simulink model "EIFANG_V1_09_09_21_RAMP_ERROR_FIXED"  (R2015a)
settings: Solver=ode4  SolverMode=MultiTasking  StartTime=0.0  StopTime=inf  FixedStep=BKIN_STEP_TIME  RelTol=1e-3
StartFcn:
  |  warndlg('Dexterit-E models cannot run under simulation. Please compile your model and run it from within Dexterit-E.');set_param(bdroot,'SimulationCommand','stop')
model workspace (MAT data in the model file):
  col_x = 1
  col_y = 2
  RADIUS_VIS = 3
  COLOR_INIT = 4
  START_TARGET_COL = 1
  DELAY_POST_TRIAL_COL = 6
  MAX_REACH_TIME_COL = 4
  DELAY_COL = 5
  E_TARGET_REACHED = 2
  BKIN_STEP_TIME = 0.00025
  BKIN_KINEMATIC_FRAME_SIZE = 400
  E_NO_EVENT = 0
  LENGTH_VIS = 5
  HEIGHT_VIS = 6
  OUT_WIDTH = 8
  IMPACT_AREA_COL = 2
  MOVING_TARGET_COL = 3
  E_AREA_REACHED = 6
  E_COLLISION = 12
  X_LOAD = 1
  Y_LOAD = 2
  RAMP = 3
  DURATION = 4
  PERTURB_COL = 7
  BGL_COL = 8
  E_UNSUCCESSFUL = 13
  FEEDBACK_TIME = 1
  HAND_FB = 2
  FIXATION_DURATION = 3
  AFTER_FIXATION = 4
  FIXATION_CROSS_ROW = 5
  DELAY_IMPACT_AREA = 6
  E_IMPACT_AREA_ON = 4
  E_CROSS_ON = 7
  E_MOVING_TARGET_ON = 10
  MAX_REACH_IMPACT_AREA = 7
  E_CROSS_OFF = 9
  OUTLINE_INIT = 7
  OUTLINE_CORRECT = 9
  OUTLINE_INCORRECT = 10
  CIRCLE_FEEDBACK_ROW = 10
  SQUARE_OUT_FEEDBACK_ROW = 8
  SQUARE_IN_FEEDBACK_ROW = 9
  E_START_TARGET = 1
  E_IMPACT_AREA = 5
  E_AREA_LEFT_CROSS = 8
  E_AREA_LEFT_TARGET = 11
  E_SUCCESSFUL = 14
  SPEED_COL = 9
  MASS_COL = 10
  ERROR_COL = 11
libraries: Video x9, KINARM_EP_loads x3, General x3, KINARM_general x3, KINARM_IO x1, simulink x1
CloseFcn:
  | rtwprivate ssgencode ModelCloseRequest b2lab2d
settings Model: ModifiedComment=chris -- Wed Feb 16 09:18:30 2005 -- Version 1.1384  ModifiedHistory=Feb 16/05 - Add error repeat, add offset ramp  ExtModeArmWhenConnect=off  ExtModeLogAll=off  Creator=Chris Grebeldinger  LastModifiedBy=obs5081
settings SolverCC: EnableConcurrentExecution=on  AutoInsertRateTranBlk=on
settings DataIOCC: LimitDataPoints=off  SignalLoggingSaveFormat=ModelDataLogs  SaveOutput=off  SaveTime=off  SignalLoggingName=sigsOut
settings OptimizationCC: BlockReduction=off  BooleanDataType=off  OptimizeBlockIOStorage=off  BufferReuse=off  GlobalBufferReuse=off  ExpressionFolding=off  ExpressionDepthLimit=2147483647  LocalBlockOutputs=off  InitFltsAndDblsToZero=on
settings DebuggingCC: SaveWithParameterizedLinksMsg=none  UnderspecifiedInitializationDetection=Classic  MergeDetectMultiDrivingBlocksExec=none  SignalResolutionControl=TryResolveAllWithWarning  MultiTaskDSMMsg=warning  FcnCallInpInsideContextMsg=UseLocalSettings  BusObjectLabelMismatch=none  StateNameClashWarn=warning  StrictBusMsg=ErrorOnBusTreatedAsVector
settings HardwareCC: ProdIntDivRoundTo=Zero  ProdEndianess=LittleEndian  ProdLongLongMode=on  ProdHWDeviceType=Generic->32-bit x86 compatible  TargetHWDeviceType=32-bit Generic
settings SFSimCC: SimCustomHeaderCode="#include \"stdlib.h\""  SFSimEcho=off  SimParseCustomCode=off
settings RTWCC: SystemTargetFile=slrt.tlc  TemplateMakefile=slrt_default_tmf  Description=Simulink Real-Time  CustomSourceCode="#include \"stdlib.h\""
settings CodeAppCC: MaxIdLength=63
settings SimulinkRealTimeCC: TargetFcnLib=ansi_tfl_tmw.mat  GeneratePreprocessorConditionals=Disable all  xPCisDownloadable=off  xPCisDefaultEnv=off

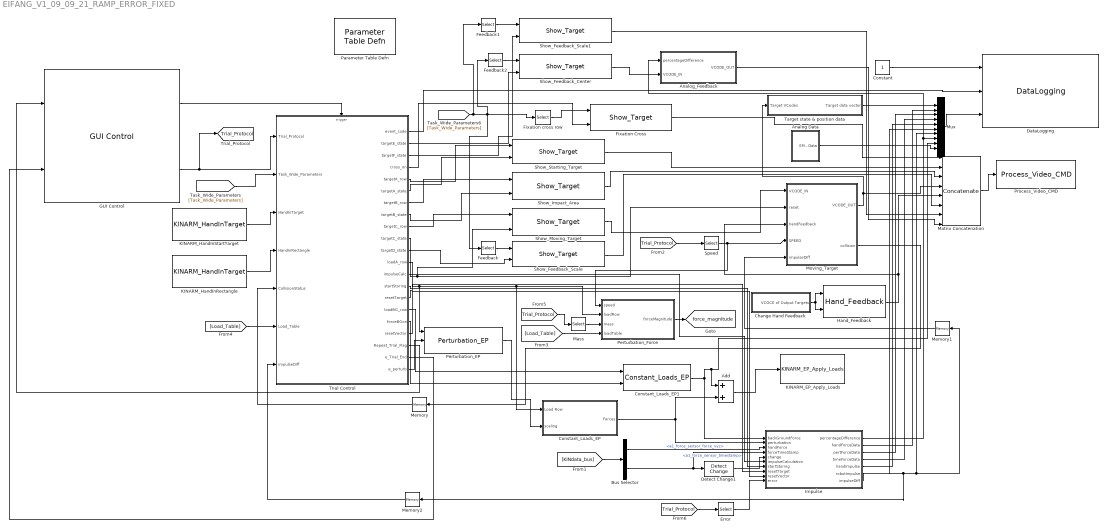
== system EIFANG_V1_09_09_21_RAMP_ERROR_FIXED ==
  Add : Sum
  Analog Data : Subsystem
  Analog_Feedback : MATLAB Function  TreatAsAtomicUnit=on
  Bus Selector : BusSelector  OutputSignals=Robot1.a1_force_sensor_force_xyz,Robot1.a1_force_sensor_timestamp
  Change Hand Feedback : Subsystem
  Constant : Constant
  Constant_Loads_EP : Subsystem  AncestorBlock=KINARM_EP_loads/Constant_Loads_EP  mask(Constant_Loads_EP){use_dom_hand=on, loadcol=[ X_LOAD Y_LOAD], source=port, scaling=1, use_LH_coord=on}
      mask prompts: use_dom_hand "Load on "arm to be assessed""; loadcol "Load Table columns [colA colB]"; source "Source for scaling"; use_LH_coord "Use left-handed coordinate frame for left-handed KINARMs"
      mask help:
      | The Constant_Loads_EP block creates constant loads on the KINARM End-Point robot in a global cartesion space, at the end-point (i.e. handle).
      |
      | Hand force (N) is calculated as:
      | Fx = A
      | Fy = B
      | (x refers to x-direction and y refers to y-direction)
      |
      | Parameters A & B in the above equations come from the Load Table, with the row determined by the "row" input to this block and the columns specified in the "Load Table columns" defined below.
      |
      | The load can be scaled by a constant internal value or a Task Program-determined external value.  (Scaling of 1 = 100%)
      mask init:
      | library = 'KINARM_EP_loads';
      | numCol = 2;
      | [inputname1, inputname2, inputname3, outputname, columntext] = loadBlockInitCommands(gcb, library, numCol);
      mask Help:
      | Used to create a force vector for applying a constant force field at the handle.
      | 
      | <H2>Library </H2>
      | KINARM EP loads
      | 
      | 
      | <H2>Description </H2>
      |  The Constant_Loads_EP block creates constant loads on the KINARM End-Point robot in a global cartesion space, at the end-point (i.e. handle).
      |  <P>
      | Force field at the fingertip (N) is calculated as: <BR>
      | Fx = A <BR>
      | Fy = B <BR>
      | (x refers to x-direction and y refers to y-direction)
      | <P>
      | For example, a y-direction force field would be A=0, B=0.5.
      | <br>For example, if the "row" input = 2, and "Load Table columns" are specifed as [1 2], then using the sample Load Table below, A = 1 and B = 0.544.
      | <br>
      | <tt>
      | __________________________<br>
      | |&nbsp;&nbsp;&nbsp;&nbsp;&nbsp;&nbsp;&nbsp;&nbsp;|Force X|Force Y|<br>
      | --------------------------<br>
      | | Load 1 |&nbsp;&nbsp;&nbsp;&nbsp;&nbsp;0 |&nbsp;&nbsp;&nbsp;&nbsp;&nbsp;0 |<br>
      | | Load 2 |&nbsp;&nbsp;&nbsp;&nbsp;&nbsp;1 | 0.544 |<br>
      | | Load 3 |&nbsp;&nbsp;&nbsp;&nbsp;-2 |&nbsp;&nbsp;&nbsp;&nbsp;&nbsp;0 |<br>
      | --------------------------<br>
      | </tt>
      | <P>
      | 
      | <P>
      | <B>row: </B> this scalar input indicates which row in the Load Table the co-efficients [A, B] will come from.
      | <P>
      | <B>Scaling: </B> this scalar input is only present if 'port' source for scaling has been chosen in the dialog box (see below).  When it is present, the actual value of the loads output from this block are scaled by this input.  For 100% of desired load, scaling=1.
      | <P>
      | <B>Forces: </B> this vector output is in global, cartesian coordinate space.  It must be wired to the KINARM_EP_Apply_Loads block to actually apply the loads to the KINARM End-Point.  This output may be added to other Force outputs from other KINARM End-Point load blocks to create a composite load.
      | <P>
      | 
      | 
      | <H2>Parameters and Dialog Box</H2>
      | <P>
      | <B>Load on "arm to be assessed":</B> this checkbox determines which arm the load is applied to. In Dexterit-E the operator selects the "arm to be assessed" using radio buttons.
      | When this box is checked the load is applied to the arm corresponding to the arm selection made by the operator in Dexterit-E.
      | When this box is unchecked the load is applied to the contralateral arm.
      | <P>
      | <B>Load Table Columns: </B> needs to be a 2x1 vector with the vector elements corresponding to the columns in the Load Table for parameters A and B.  If a parameter is not going to be in the Load Table, then the value 0 should be used in the "Load Table Columns" vector  (e.g. if only y-direction loads are specified in the Load Table, and the y-direction load is in column 2, then the "Load Table Columns" vector should be [0 2], which indicates that parameter A is not specified in the Load Table and so A is set =0).
      | <P>
      | <B>Source for scaling: </B> refers to the source for scaling of the load.  If the source is dialog, then a Scaling option appears in the Dialog box.  If the source is port, then a new input appears to this Simulink block.  For loads that are always on, use a dialog scale with the value set to 1.  For loads that need to be controlled by the Task Program machine (e.g. to turn them on or off) or by an external block (e.g. to ramp up a load), use a port source for the scaling.
      | <P>
      | <B>Scaling: </B>  this dialog input is only present if 'dialog' source for scaling has been chosen in the dialog box.  When it is present, the actual value of the loads output from this block are scaled by this input.  For 100% of desired load, scaling=1.
      | <P>
      | <B>Use left-handed coordinate system for left-handed KINARMs.  </B> This checkbox only affects left-handed KINARMs.  If checked, then a left-handed coordinate system is used for left-handed KINARMs (i.e. x is positive to the left).  If unchecked, then a right-handed coordinate system is used.  Right-handed KINARMs always use a right-handed coordinate frame (i.e. x is positive to the right).
      | <P>
      | 
      | 
      | <H2>Related Blocks </H2>
      | KINARM_EP_Apply_Loads<BR>
      | Perturbation_EP
      mask Callback loadcol:
      | %%%%
      | % Because of bugs iN R2007, R2010a and R2013a (which have been reported to Mathworks), the following code
      | % is required here because in the Initialization Section it will ONLY correctly update those Mask Parameters that are hidden
      | % when the OK button is clicked (NOTE: the initialization code will correctly update all Mask Parameters when the Apply button
      | % is clicked, the bug is that it should also update everything when the OK button is clicked in the absence of an Apply click)
      | %
      | % Adding a set_param call which updates one of the mask parameters will call the initialization code to run, which "avoids"
      | % this bug. This code should be removed once Mathworks has fixed this bug.
      | 
      | temp = get_param(gcb, 'loadcol');
      | set_param(gcb, 'loadcol', temp);
      mask TypeOptions source: dialog | port
      mask Callback source:
      | sourceStr=get_param(gcb,'source');
      | vis=get_param(gcb,'MaskVisibilities');
      | 
      | if strmatch(sourceStr, 'dialog')
      | 	vis{4}='on';
      | else
      | 	vis{4}='off';
      | end
      | 
      | set_param(gcb,'MaskVisibilities',vis);
      mask Display: disp(columntext); port_label('output',1,outputname); port_label('input',1, inputname1); port_label('input',2, inputname2);
  Constant_Loads_EP1 : KINARM_EP_loads/Constant_Loads_EP  use_dom_hand=on  loadcol=[X_LOAD Y_LOAD]  source=port  scaling=1  use_LH_coord=on
  DataLogging : General/DataLogging  log_event_codes=on  log_analog_inputs=on  show_time_remaining=off  ecat_include=on
  Detect Change1 : simulink/Logic and Bit Operations/Detect Change  vinit=0  InputProcessing=Inherited  OutDataTypeStr=boolean
  Error : Selector  Indices=ERROR_COL
  Feedback : Selector  Indices=SQUARE_OUT_FEEDBACK_ROW
  Feedback1 : Selector  Indices=SQUARE_IN_FEEDBACK_ROW
  Feedback2 : Selector  Indices=CIRCLE_FEEDBACK_ROW
  Fixation Cross : Video/Show_Target  target_type=Circle  num_states=1  attribcol1=[COLOR_INIT 0 0 RADIUS_VIS]  attribcol2=[0 0 0 0]  attribcol3=[0 0 0 0]  attribcol4=[0 0 0 0]  attribcol5=[0 0 0 0]  stateindices_padding=[0 0 0 0 0 0 0;0 0 0 0 0 0 0;0 0 0 0 0 0 0;0 0 0 0 0 0 0;0 0 0 0 0 0 0]  source=dialog  opacity=100  target_display=Both subject and operator displays  num_col=4
  Fixation cross row : Selector  Indices=FIXATION_CROSS_ROW
  GUI Control : General/GUI Control  task_version=1.0  show_repeat_trial_flag=on  use_custom_tp=off  target_type_str=Circle  Target_Type=1  XYcols=[1 2]  Vcols=3  Lcols=4  indices_padding=[0 0 0 0;0 0 0 0]  target_table_rows=64  load_table_rows=20  tp_table_rows=100
  Hand_Feedback : KINARM_general/Hand_Feedback  feedback_cntl_src=style and status
  Impulse : MATLAB Function  TreatAsAtomicUnit=on
  KINARM_EP_Apply_Loads : KINARM_EP_loads/KINARM_EP_Apply_Loads  up_duration=500  down_duration=500  max_force=15
  KINARM_HandInRectangle : KINARM_general/KINARM_HandInTarget  use_dominant_hand=on  target_type=Rectangle  num_states=1  attribcol1=[LENGTH_VIS HEIGHT_VIS 0]  attribcol2=[0 0 0]  attribcol3=[0 0 0]  attribcol4=[0 0 0]  attribcol5=[0 0 0]
  KINARM_HandInStartTarget : KINARM_general/KINARM_HandInTarget  use_dominant_hand=on  target_type=Rectangle  num_states=1  attribcol1=[LENGTH_VIS HEIGHT_VIS 0]  attribcol2=[0 0 0]  attribcol3=[0 0 0]  attribcol4=[0 0 0]  attribcol5=[0 0 0]
  Mass : Selector  Indices=MASS_COL
  Matrix Concatenation : Concatenate  NumInputs=8  Mode=Multidimensional array
  Memory : Memory
  Memory1 : Memory
  Memory2 : Memory
  Moving_Target : MATLAB Function  TreatAsAtomicUnit=on
  Mux : Mux  Inputs=10
  Parameter Table Defn : General/Parameter Table Defn  ShowInLibBrowser=0
  Perturbation_EP : KINARM_EP_loads/Perturbation_EP  loadcol=[RAMP DURATION RAMP]
  Perturbation_Force : MATLAB Function  TreatAsAtomicUnit=on
  Process_Video_CMD : Video/Process_Video_CMD  video_delay=50
  Show_Feedback_Center : Video/Show_Target  target_type=Rectangle  num_states=1  attribcol1=[COLOR_INIT OUTLINE_INIT OUT_WIDTH LENGTH_VIS HEIGHT_VIS 0]  attribcol2=[0 0 0 0 0 0]  attribcol3=[0 0 0 0 0 0]  attribcol4=[0 0 0 0 0 0]  attribcol5=[0 0 0 0 0 0]  stateindices_padding=[0 0 0 0 0;0 0 0 0 0;0 0 0 0 0;0 0 0 0 0;0 0 0 0 0]  source=dialog  opacity=100  target_display=Both subject and operator displays  num_col=6
  Show_Feedback_Scale : Video/Show_Target  target_type=Rectangle  num_states=1  attribcol1=[COLOR_INIT OUTLINE_INIT OUT_WIDTH LENGTH_VIS HEIGHT_VIS 0]  attribcol2=[0 0 0 0 0 0]  attribcol3=[0 0 0 0 0 0]  attribcol4=[0 0 0 0 0 0]  attribcol5=[0 0 0 0 0 0]  stateindices_padding=[0 0 0 0 0;0 0 0 0 0;0 0 0 0 0;0 0 0 0 0;0 0 0 0 0]  source=dialog  opacity=100  target_display=Both subject and operator displays  num_col=6
  Show_Feedback_Scale1 : Video/Show_Target  target_type=Rectangle  num_states=1  attribcol1=[COLOR_INIT OUTLINE_INIT OUT_WIDTH LENGTH_VIS HEIGHT_VIS 0]  attribcol2=[0 0 0 0 0 0]  attribcol3=[0 0 0 0 0 0]  attribcol4=[0 0 0 0 0 0]  attribcol5=[0 0 0 0 0 0]  stateindices_padding=[0 0 0 0 0;0 0 0 0 0;0 0 0 0 0;0 0 0 0 0;0 0 0 0 0]  source=dialog  opacity=100  target_display=Both subject and operator displays  num_col=6
  Show_Impact_Area : Video/Show_Target  target_type=Rectangle  num_states=3  attribcol1=[0 OUTLINE_INIT OUT_WIDTH LENGTH_VIS HEIGHT_VIS 0]  attribcol2=[0 OUTLINE_CORRECT OUT_WIDTH LENGTH_VIS HEIGHT_VIS 0]  attribcol3=[0 OUTLINE_INCORRECT OUT_WIDTH LENGTH_VIS HEIGHT_VIS 0]  attribcol4=[0 0 0 0 0 0]  attribcol5=[0 0 0 0 0 0]  stateindices_padding=[0 0 0 0 0;0 0 0 0 0;0 0 0 0 0;0 0 0 0 0;0 0 0 0 0]  source=dialog  opacity=100  target_display=Both subject and operator displays  num_col=6
  Show_Moving_Target : Video/Show_Target  target_type=Circle  num_states=1  attribcol1=[COLOR_INIT 0 0 RADIUS_VIS]  attribcol2=[0 0 0 0]  attribcol3=[0 0 0 0]  attribcol4=[0 0 0 0]  attribcol5=[0 0 0 0]  stateindices_padding=[0 0 0 0 0 0 0;0 0 0 0 0 0 0;0 0 0 0 0 0 0;0 0 0 0 0 0 0;0 0 0 0 0 0 0]  source=dialog  opacity=100  target_display=Both subject and operator displays  num_col=4
  Show_Starting_Target : Video/Show_Target  target_type=Rectangle  num_states=1  attribcol1=[COLOR_INIT OUTLINE_INIT OUT_WIDTH LENGTH_VIS HEIGHT_VIS 0]  attribcol2=[0 0 0 0 0 0]  attribcol3=[0 0 0 0 0 0]  attribcol4=[0 0 0 0 0 0]  attribcol5=[0 0 0 0 0 0]  stateindices_padding=[0 0 0 0 0;0 0 0 0 0;0 0 0 0 0;0 0 0 0 0;0 0 0 0 0]  source=dialog  opacity=100  target_display=Both subject and operator displays  num_col=6
  Speed : Selector  Indices=SPEED_COL
  Target state & position data : Subsystem
  Trial Control : Stateflow chart  TreatAsAtomicUnit=on
  tag scope: Trial_Protocol=global, force_magnitude=global
  wires:
  Trial Control/20(e_Trial_End) -> GUI Control/2
  GUI Control/1 -> Trial Control/Trigger
  Trial Control/6(targetA_state) -> Show_Starting_Target/2
  Trial Control/5(targetA_row) -> Show_Starting_Target/1
  Matrix Concatenation/1 -> Process_Video_CMD/1
  Trial Control/1(event_code) -> DataLogging/2
  Show_Starting_Target/1 -> Matrix Concatenation/2
  Constant/1 -> DataLogging/1
  GUI Control/2 -> [Trial_Protocol], Trial Control/1(Trial_Protocol)
  KINARM_HandInStartTarget/1 -> Trial Control/3(HandInTarget)
  Trial Control/7(targetB_row) -> Show_Impact_Area/1
  Trial Control/8(targetB_state) -> Show_Impact_Area/2
  Show_Impact_Area/1 -> Matrix Concatenation/3
  Trial Control/10(targetC_state) -> Moving_Target/2(reset), Show_Moving_Target/2
  Trial Control/9(targetC_row) -> Show_Moving_Target/1
  Show_Moving_Target/1 -> Moving_Target/1(VCODE_IN)
  Hand_Feedback/1 -> Matrix Concatenation/5, Moving_Target/3(handFeedback)
  Moving_Target/1(VCODE_OUT) -> Matrix Concatenation/4, Target state & position data/1(Target VCodes)
  KINARM_HandInRectangle/1 -> Trial Control/4(HandInRectangle)
  Moving_Target/2(collision) -> Memory/1
  Memory/1 -> Trial Control/5(CollisionStatus)
  [Trial_Protocol] -> Speed/1
  Perturbation_EP/1 -> Constant_Loads_EP/2(scaling)
  Trial Control/12(loadA_row) -> Perturbation_Force/2(loadRow), Constant_Loads_EP/1(Load Row), Perturbation_EP/1
  Trial Control/21(e_perturb) -> Perturbation_EP/2
  [KINdata_bus] -> Bus Selector/1
  Target state & position data/1(Target data vector) -> Mux/1
  [Load_Table] -> Perturbation_Force/4(loadTable)
  Perturbation_Force/1(forceMagnitude) -> [force_magnitude]
  Bus Selector/1 -> Impulse/3(handForce)  "<a1_force_sensor_force_xyz>"
  Constant_Loads_EP/1(Forces) -> Add/2, Impulse/2(perturbation)
  Mux/1 -> DataLogging/3
  Detect Change1/1 -> Impulse/5(change)
  Bus Selector/2 -> Detect Change1/1, Impulse/4(forceTimeStamp)  "<a1_force_sensor_timestamp>"
  Trial Control/13(impulseCalc) -> Impulse/6(impulseCalculation)
  Trial Control/14(startStoring) -> Impulse/7(startStoring)
  Impulse/2(handForceData) -> Mux/2
  Impulse/4(timeForceData) -> Mux/4
  Impulse/5(handImpulse) -> Mux/5
  Impulse/6(robotImpulse) -> Mux/6
  [Load_Table] -> Trial Control/6(Load_Table)
  Impulse/3(pertForceData) -> Mux/3
  Impulse/7(impulseDiff) -> Mux/7, Memory1/1, Memory2/1
  Memory1/1 -> Moving_Target/5(impulseDiff)
  Trial Control/15(resetTarget) -> Impulse/8(resetTarget)
  Add/1 -> KINARM_EP_Apply_Loads/1
  Constant_Loads_EP1/1 -> Mux/9, Add/1, Impulse/1(backGroundForce)
  Trial Control/16(loadBG_row) -> Constant_Loads_EP1/1
  Trial Control/17(forceBGon) -> Constant_Loads_EP1/2
  Trial Control/18(resetVector) -> Impulse/9(resetVector)
  [Task_Wide_Parameters] -> Trial Control/2(Task_Wide_Parameters)
  Memory2/1 -> Trial Control/7(impulseDiff)
  Change Hand Feedback/1(VCOCE of Output Targets) -> Hand_Feedback/2, Hand_Feedback/1
  Trial Control/4(cross_on) -> Fixation Cross/2
  [Task_Wide_Parameters] -> Feedback1/1, Feedback/1, Fixation cross row/1, Feedback2/1
  Fixation cross row/1 -> Fixation Cross/1
  Fixation Cross/1 -> Matrix Concatenation/1
  Analog Data/1(EMG Data) -> Mux/10
  Feedback/1 -> Show_Feedback_Scale/1
  Trial Control/11(targetD_state) -> Show_Feedback_Scale/2
  Show_Feedback_Scale/1 -> Matrix Concatenation/6
  Trial Control/2(targetE_state) -> Show_Feedback_Center/2
  Feedback2/1 -> Show_Feedback_Center/1
  Analog_Feedback/1(VCODE_OUT) -> Matrix Concatenation/8
  Trial Control/3(targetF_state) -> Show_Feedback_Scale1/2
  Feedback1/1 -> Show_Feedback_Scale1/1
  Show_Feedback_Scale1/1 -> Matrix Concatenation/7
  Impulse/1(percentageDifference) -> Mux/8, Analog_Feedback/1(percentageDifference)
  Show_Feedback_Center/1 -> Analog_Feedback/2(VCODE_IN)
  Speed/1 -> Perturbation_Force/1(speed), Moving_Target/4(SPEED)
  [Trial_Protocol] -> Mass/1
  Mass/1 -> Perturbation_Force/3(mass)
  Trial Control/19(Repeat_Trial_Flag) -> GUI Control/1
  [Trial_Protocol] -> Error/1
  Error/1 -> Impulse/10(error)

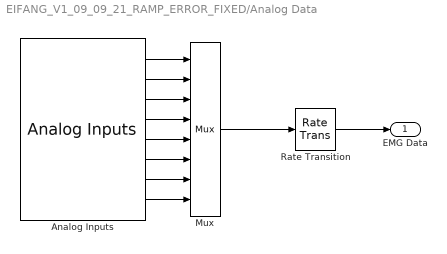
== system EIFANG_V1_09_09_21_RAMP_ERROR_FIXED/Analog Data ==
  Analog Inputs : KINARM_IO/Analog Inputs  channel=[1:8]  range=[5]  coupling=[0]  scantime6071e=1.28e-5  scantime6229=5e-6  sampletime=0.001  slot=-1  oscantime6071e=0
  Mux : Mux  Inputs=8
  Rate Transition : RateTransition
  EMG Data : Outport
  wires:
  Mux/1 -> Rate Transition/1
  Analog Inputs/5 -> Mux/5
  Analog Inputs/6 -> Mux/6
  Analog Inputs/4 -> Mux/4
  Analog Inputs/2 -> Mux/2
  Analog Inputs/1 -> Mux/1
  Analog Inputs/3 -> Mux/3
  Analog Inputs/8 -> Mux/8
  Analog Inputs/7 -> Mux/7
  Rate Transition/1 -> EMG Data/1

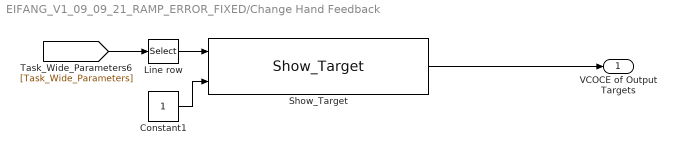
== system EIFANG_V1_09_09_21_RAMP_ERROR_FIXED/Change Hand Feedback ==
  Constant1 : Constant
  Line row : Selector  Indices=HAND_FB
  Show_Target : Video/Show_Target  target_type=Rectangle  num_states=1  attribcol1=[COLOR_INIT COLOR_INIT RADIUS_VIS LENGTH_VIS HEIGHT_VIS 0]  attribcol2=[0 0 0 0 0 0]  attribcol3=[0 0 0 0 0 0]  attribcol4=[0 0 0 0 0 0]  attribcol5=[0 0 0 0 0 0]  stateindices_padding=[0 0 0 0 0;0 0 0 0 0;0 0 0 0 0;0 0 0 0 0;0 0 0 0 0]  source=dialog  opacity=100  target_display=Both subject and operator displays  num_col=6
  VCOCE of Output Targets : Outport
  wires:
  Constant1/1 -> Show_Target/2
  Show_Target/1 -> VCOCE of Output Targets/1
  [Task_Wide_Parameters] -> Line row/1
  Line row/1 -> Show_Target/1

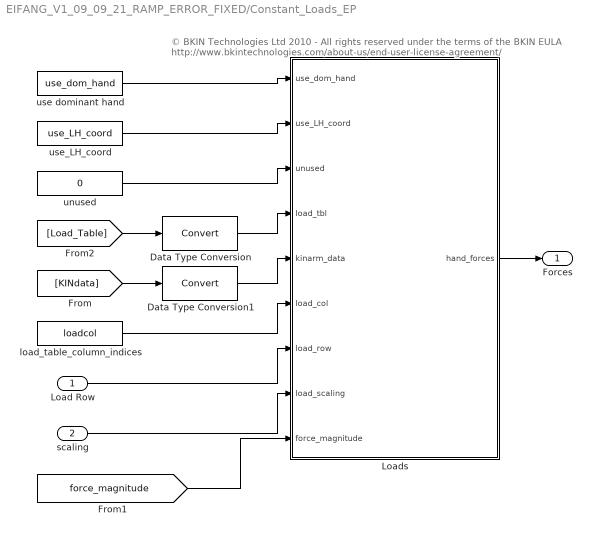
== system EIFANG_V1_09_09_21_RAMP_ERROR_FIXED/Constant_Loads_EP ==
  note: © BKIN Technologies Ltd 2010  - All rights reserved under the terms of the BKIN EULA
      | http://www.bkintechnologies.com/about-us/end-user-license-agreement/
  Load Row : Inport
  scaling : Inport  Port=2
  Data Type Conversion : DataTypeConversion
  Data Type Conversion1 : DataTypeConversion
  Loads : MATLAB Function  TreatAsAtomicUnit=on
  load_table_column_indices : Constant  Value=loadcol
  unused : Constant  Value=0
  use dominant hand : Constant  Value=use_dom_hand
  use_LH_coord : Constant  Value=use_LH_coord
  Forces : Outport
  wires:
  Loads/1(hand_forces) -> Forces/1
  use_LH_coord/1 -> Loads/2(use_LH_coord)
  unused/1 -> Loads/3(unused)
  load_table_column_indices/1 -> Loads/6(load_col)
  Load Row/1 -> Loads/7(load_row)
  [KINdata] -> Data Type Conversion1/1
  [Load_Table] -> Data Type Conversion/1
  use dominant hand/1 -> Loads/1(use_dom_hand)
  Data Type Conversion/1 -> Loads/4(load_tbl)
  Data Type Conversion1/1 -> Loads/5(kinarm_data)
  scaling/1 -> Loads/8(load_scaling)
  [force_magnitude] -> Loads/9(force_magnitude)

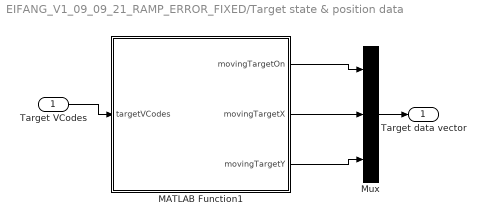
== system EIFANG_V1_09_09_21_RAMP_ERROR_FIXED/Target state & position data ==
  Target VCodes : Inport
  MATLAB Function1 : MATLAB Function  TreatAsAtomicUnit=on
  Mux : Mux  Inputs=3
  Target data vector : Outport
  wires:
  Mux/1 -> Target data vector/1
  Target VCodes/1 -> MATLAB Function1/1(targetVCodes)
  MATLAB Function1/1(movingTargetOn) -> Mux/1
  MATLAB Function1/2(movingTargetX) -> Mux/2
  MATLAB Function1/3(movingTargetY) -> Mux/3

== matlab function EIFANG_V1_09_09_21_RAMP_ERROR_FIXED/Moving_Target ==
  data: VCODE_IN input; VCODE_OUT output; reset input; handFeedback input; SPEED input; collision output; impulseDiff input
function [VCODE_OUT,collision]= fcn(VCODE_IN, reset, handFeedback, SPEED,impulseDiff)
%This function changes the Y position of the target so it moves down in a
%straight line
speed = SPEED/4000; % The sampling rate of the task program is 4000 and therefore we are doing the division

VCODE_OUT = VCODE_IN;
collision = 0;

%This part chooses a random speed for each trial between the max and min
%inputed by the user
persistent yOffset yOffsetReturn k position


if isempty(yOffset)
    yOffset = 0;
    yOffsetReturn = 0;
    k = 1;
    position = 0;
end

yOffset = yOffset - speed;


%This part changes the VCODE to make the target move
if isempty(yOffset) || reset == 0
    yOffset = 0;
    yOffsetReturn = 0;
    k = 1;
    position = 0;
end
% if yOffset + VCODE_OUT(4) < 0
%     yOffset = -VCODE_OUT(4);
%     collision = 2; %abort trial
% end

%This part determines what happens with the target after the collision
if impulseDiff ~= 0
    if impulseDiff == 2 
        if k == 1
            position = yOffset;
            k = 2;
        end
        VCODE_OUT(4) = VCODE_OUT(4) + position; %target stops
    elseif impulseDiff == 3
        if k == 1
            position = yOffset;
            k = 2;
        end
        yOffsetReturn = yOffsetReturn + speed;
        VCODE_OUT(4) = VCODE_OUT(4) + position + yOffsetReturn; %target bounces back
    elseif impulseDiff == 1
        VCODE_OUT(4) = VCODE_OUT(4) + yOffset; %target keeps moving
    end
elseif impulseDiff == 0
VCODE_OUT(4)= VCODE_OUT(4) + yOffset; 
end

%This part determines when the collision happens
distanceY=abs(VCODE_OUT(4)-handFeedback(1,4)); 
distanceX=abs(VCODE_OUT(3)-handFeedback(1,3));

if distanceY < 0.01 && distanceX < 0.01
    collision = 1; %a collision happened
end

       
end

== stateflow chart EIFANG_V1_09_09_21_RAMP_ERROR_FIXED/Trial Control ==
  state MainTrial
    state ShowStartingTarget/
      // Turn on first target and wait for a specified time or until the hand is in the target.
      targetA_row = Trial_Protocol[START_TARGET_COL];
      targetA_state = 1;
      targetB_state = 0;
      targetC_state = 0;
      targetD_state = 0;
      targetE_state = 0;
      targetF_state = 0;
      startStoring = 0;
      impulseCalc = 0;
      resetTarget = 0;
      forceBGon = 0;
      resetVector = 0;
      cross_on = 0;
      Repeat_Trial_Flag = 0;
      loadBG_row = Trial_Protocol[BGL_COL];
      tickCount = Trial_Protocol[MAX_REACH_TIME_COL] ;
      loadA_row = Trial_Protocol[PERTURB_COL];
    state StayAtStartingTarget/
      // Log an event that target was reached and then wait for a specified time.
      event_code = E_TARGET_REACHED;
      tickCount = Trial_Protocol[DELAY_COL] ;
    state UnsuccessfulTrial4/
      event_code = E_START_TARGET;
      Repeat_Trial_Flag = 1;
    state ShowImpactArea/
      targetB_row = Trial_Protocol[IMPACT_AREA_COL];
      targetB_state = 1;
      event_code = E_IMPACT_AREA_ON;
    state HandInImpactArea/
      event_code = E_AREA_REACHED;
      targetA_state = 0;
      forceBGon = 1;
    state HandOutImpactArea/
      event_code = E_AREA_LEFT_CROSS;
      Repeat_Trial_Flag = 1;
    state CrossOn/
      cross_on = 1;
      event_code = E_CROSS_ON;
    state UnsuccessfulTrial3/
      event_code = E_IMPACT_AREA;
      Repeat_Trial_Flag = 1;
    state CrossOff/
      cross_on = 0;
      event_code=E_CROSS_OFF;
    state ShowMovingTarget/
      // Show moving traget
      targetC_row = Trial_Protocol[MOVING_TARGET_COL];
      targetC_state = 1;
      event_code = E_MOVING_TARGET_ON;
    state HandOutImpactArea1/
      event_code = E_AREA_LEFT_TARGET;
      Repeat_Trial_Flag = 1;
    state ResetImpactVector/
      resetVector = 1;
    state Collision/
      resetVector = 0;
      startStoring=1;
      event_code = E_COLLISION;
      tickCount = Load_Table[loadA_row][RAMP]*2 + Load_Table[loadA_row][DURATION];
      e_perturb;
    state StartImpulse/
      startStoring = 0;
      impulseCalc = 1;
    state UnsuccessfulTrial/
      event_code = E_UNSUCCESSFUL;
    state FinishImpulse/
      impulseCalc = 0;
    state ColorFeedback/
      targetB_state = 2;
      targetD_state = 1;
      targetE_state = 1;
      targetF_state = 1;
      event_code = E_SUCCESSFUL;
    state ColorFeedback1/
      targetB_state = 3;
      targetD_state = 1;
      targetE_state = 1;
      targetF_state = 1;
    state EndOfTrial/
      // Turn off the target, set the post-trial delay
      targetB_state = 0;
      targetC_state = 0;
      targetD_state = 0;
      targetE_state = 0;
      targetF_state = 0;
      resetTarget  = 1;
      forceBGon = 0;
      tickCount = Trial_Protocol[DELAY_POST_TRIAL_COL];
    ShowStartingTarget -> StayAtStartingTarget [order 2] : // is the hand in the target?
        | // value == 0 indicates "not in target"
        | // value == 1 indicates "in target"
        | [HandInTarget[targetA_row] == 1]
    ShowStartingTarget -> UnsuccessfulTrial4 [order 1] : // has a a specified period of
        | // time occured?
        | after(tickCount, e_clk)
    StayAtStartingTarget -> ShowImpactArea : // has a a specified period of time occured?
        | after(tickCount, e_clk)
    ShowImpactArea -> UnsuccessfulTrial3 [order 2] : after(Task_Wide_Parameters[MAX_REACH_IMPACT_AREA], e_clk)
    UnsuccessfulTrial4 -> EndOfTrial
    ShowImpactArea -> HandInImpactArea [order 1] : // is the hand in the impact area?
        | [HandInRectangle[targetB_row] == 1]
    HandInImpactArea -> CrossOn : after(Task_Wide_Parameters[DELAY_IMPACT_AREA], e_clk)
    CrossOn -> HandOutImpactArea [order 1] : // is the hand out the impact area?
        | [HandInRectangle[targetB_row] == 0]
    HandOutImpactArea -> EndOfTrial
    CrossOn -> CrossOff [order 2] : after(Task_Wide_Parameters[FIXATION_DURATION], e_clk)
    CrossOff -> ShowMovingTarget : after(Task_Wide_Parameters[AFTER_FIXATION], e_clk)
    UnsuccessfulTrial3 -> EndOfTrial
    ShowMovingTarget -> EndOfTrial [order 3] : [CollisionStatus == 2]
    ShowMovingTarget -> HandOutImpactArea1 [order 2] : // is the hand out the impact area?
        | [HandInRectangle[targetB_row] == 0]
    HandOutImpactArea1 -> EndOfTrial
    ShowMovingTarget -> ResetImpactVector [order 1] : // hand and target collided?
        | [CollisionStatus == 1]
    ResetImpactVector -> Collision
    Collision -> StartImpulse : after(tickCount,e_clk)
    StartImpulse -> FinishImpulse
    FinishImpulse -> UnsuccessfulTrial [order 2] : [impulseDiff == 1 || impulseDiff == 3]
    FinishImpulse -> ColorFeedback [order 1] : [impulseDiff == 2]
    UnsuccessfulTrial -> ColorFeedback1
    ColorFeedback -> EndOfTrial : after(Task_Wide_Parameters[FEEDBACK_TIME], e_clk)
    ColorFeedback1 -> EndOfTrial : after(Task_Wide_Parameters[FEEDBACK_TIME], e_clk)
  state Initialiize/
    // If there was something to initialize
    // do it here
  state Inter_Trial_State/
    // Turn off target, reset the event code, and send the
    //e_Trial_End Stateflow event to indicate that the trial is over.
    event_code = 0;
    targetA_state = 0;
    e_Trial_End;
  (default) -> Initialiize
  Initialiize -> ShowStartingTarget
  Inter_Trial_State -> ShowStartingTarget : // has a a specified period of
      | // time occured?
      | after(tickCount, e_clk)
  MainTrial -> Inter_Trial_State : e_ExitTrialNow/
      | tickCount = 1;
      | // e_ExitTrialNow event occurs if the
      | // Dex pause is pressed by the operator
  EndOfTrial -> Inter_Trial_State
  data: event_code output uint16 [0..] =0; targetE_state output double; targetF_state output double; cross_on output double; targetA_row output [1..32]; targetA_state output double; tickCount local double; Trial_Protocol input double; Task_Wide_Parameters input double; HandInTarget input double; targetB_row output double; targetB_state output double; targetC_row output double; targetC_state output double; targetD_state output double; HandInRectangle input double; CollisionStatus input double; loadA_row output; impulseCalc output boolean; startStoring output double; Load_Table input double; resetTarget output double; loadBG_row output double; forceBGon output double; resetVector output double; impulseDiff input double; Repeat_Trial_Flag output double
  data targetA_row settings: description=index of the row currently being used in the TargetTable
  events: e_clk input RISING_EDGE_EVENT; e_ExitTrialNow input EITHER_EDGE_EVENT; e_Trial_End output EITHER_EDGE_EVENT; e_perturb output EITHER_EDGE_EVENT

== matlab function EIFANG_V1_09_09_21_RAMP_ERROR_FIXED/Analog_Feedback ==
  data: percentageDifference input; VCODE_OUT output; VCODE_IN input
function VCODE_OUT = fcn(percentageDifference,VCODE_IN)
%This function changes the X position of the circle for the visual analog
%scale for the feedback

VCODE_OUT = VCODE_IN;

persistent feedbackPosition

if isempty(feedbackPosition)
    feedbackPosition = 0;
end
initialPosition = 0;
if percentageDifference ~= 100
    feedbackPosition = percentageDifference/100;    
end

feedbackPosition = feedbackPosition + initialPosition;
VCODE_OUT(3) = VCODE_OUT(3) + feedbackPosition;

end

== matlab function EIFANG_V1_09_09_21_RAMP_ERROR_FIXED/Impulse ==
  data: percentageDifference output; backGroundForce input; handForceData output; pertForceData output; timeForceData output; handImpulse output; perturbation input size=[1 4]; handForce input; forceTimeStamp input; change input; robotImpulse output; impulseDiff output; impulseCalculation input; startStoring input; resetTarget input; resetVector input; error input
function [percentageDifference,handForceData,pertForceData,timeForceData,handImpulse,robotImpulse,impulseDiff] = fcn(backGroundForce,perturbation,handForce,forceTimeStamp,change,impulseCalculation,startStoring,resetTarget,resetVector,error)
%This function calculates hand and robot's impulse

persistent k handForceImpulse perturbationYimpulse forceTime impulseDifference

handImpulse=0;
robotImpulse=0;
percentageDifference=100; %The 100 is any value that this variable will never have. 0 doesn't work because the actual difference can be 0.

if isempty(k)
    k = 1;
    handForceImpulse = zeros(1,480); 
    perturbationYimpulse = zeros(1,480);
    forceTime = zeros(1,480);
    impulseDifference = 0;
end

if resetVector == 1
    handImpulse = 0;
    robotImpulse = 0;
    k = 1;
    handForceImpulse = zeros(1,480); 
    perturbationYimpulse = zeros(1,480);
    forceTime = zeros(1,480);
    impulseDifference = 0;
end

if startStoring == 1 && change == 1
    %add to impulse vectors
    k=k+1;
    handForceImpulse(k) = handForce(2)+backGroundForce(2);
    perturbationYimpulse(k) = perturbation(2);
    forceTime(k) = forceTimeStamp;
end

j = k;
handForceData=handForceImpulse(k);
pertForceData=perturbationYimpulse(k);
timeForceData=forceTime(k);

if impulseCalculation == 1
    handForcefullimpulse = handForceImpulse;
    perturbYfullimpulse = perturbationYimpulse;
    forceTimeImpulse = forceTime;
   
    handForceImpulse(k) = 0;
    perturbationYimpulse(k) = 0;
    forceTime(k) = 0;
    k = 1;
    
    %calculate impulse
    handImpulse = trapz(forceTimeImpulse(forceTimeImpulse~=0),handForcefullimpulse(handForcefullimpulse~=0));
    robotImpulse = trapz(forceTimeImpulse(forceTimeImpulse~=0),perturbYfullimpulse(perturbYfullimpulse~=0));
    handImpulsePerc = handImpulse*100/abs(robotImpulse);
    percentageDifference = handImpulsePerc-100;
    
    robotImpulseMin = (abs(robotImpulse)*(100-error))/100;
    robotImpulseMax = (abs(robotImpulse)*(100+error))/100;
    if handImpulse < robotImpulseMin
        impulseDifference = 1; %target should keep moving
    elseif handImpulse > robotImpulseMax
        impulseDifference = 3; %target should bounce back
    else
        impulseDifference = 2; %target should stop
    end
    
    
end
impulseDiff = impulseDifference;
if resetTarget == 1
    impulseDifference = 0;
end

end

== matlab function EIFANG_V1_09_09_21_RAMP_ERROR_FIXED/Target state & position data/MATLAB Function1 ==
  data: targetVCodes input; movingTargetOn output; movingTargetX output; movingTargetY output
%This function extracts data to be saved from the target VCode matrix
%Returns a vector of doubles.

function [movingTargetOn,movingTargetX,movingTargetY] = extractDataChannels(targetVCodes)
%#codegen
    onOff = targetVCodes(:,2);
    onOff = typecast(onOff, 'double');
    xPositions = targetVCodes(:,3);
    xPositions = typecast(xPositions, 'double');
    yPositions = targetVCodes(:,4);
    yPositions = typecast(yPositions, 'double');
    
    movingTargetOn = onOff(1);
    movingTargetX = xPositions(1);
    movingTargetY = yPositions(1);
    
end

== matlab function EIFANG_V1_09_09_21_RAMP_ERROR_FIXED/Perturbation_Force ==
  data: speed input; loadRow input; mass input; loadTable input; forceMagnitude output
function forceMagnitude = fcn(speed,loadRow,mass,loadTable)
%#This function determines the perturbation force based on the velocity of each trial
%mass=2.32;
%mass=2;
ramp=loadTable(loadRow,3);
hold=loadTable(loadRow,4);
perturbationTime=ramp+hold;
forceMagnitude=-((mass*speed)/perturbationTime)*1000;
end

== matlab function EIFANG_V1_09_09_21_RAMP_ERROR_FIXED/Constant_Loads_EP/Loads ==
  settings: fimath=|
      | fimath(...
      | 'RoundMode', 'floor',...
      | 'OverflowMode', 'wrap',...
      | 'ProductMode', 'KeepLSB', 'ProductWordLength', 32,...
      | 'SumMode', 'KeepLSB', 'SumWordLength', 32,...
      | 'CastBeforeSum', false)
  data: hand_forces output; use_dom_hand input; use_LH_coord input; unused input; load_tbl input; kinarm_data input; load_col input; load_row input; load_scaling input; force_magnitude input
function hand_forces = const_loads(use_dom_hand, use_LH_coord, unused, load_tbl, kinarm_data, load_col, load_row, load_scaling,force_magnitude)
%
% CONSTANT FORCE FIELD 
%
% revision 1, Nov 5, 2005
%

% kinarm_data indicies
ORIENT_index = 6;		% 1=right	2=left

% by default, all loads are zeroed
hand_forces = [0,0,0,0];

%determine which arm to apply the load to
dominant_hand=kinarm_data(3,1);						%kinarm_data(3,1) tells which arm is the dominant arm
if use_dom_hand==1
	loading_arm=dominant_hand;
else
	loading_arm=3-dominant_hand;
end

if load_row > 0 && load_row <= size(load_tbl,1)
	CA=0;	CB=0;			%default values
	% global frame force field coefficients    
	if load_col(1)>0
		CA = load_tbl( load_row, load_col(1));
	end
	if load_col(2)>0
		CB = load_tbl( load_row, load_col(2));
	end
	% calculate force field force components
	if use_LH_coord==1 && kinarm_data( loading_arm, ORIENT_index )==2
    	hand_forces(1+2*(loading_arm-1))=-CA;			%hand x-direction force (LH coordinate)
    else
    	hand_forces(1+2*(loading_arm-1))=CA;			%hand x-direction force
    end        
	hand_forces(2+2*(loading_arm-1))=CB;			%hand y-direction force
   
end

%Overwrite perturbation Y magnitude
hand_forces(2) = hand_forces(2) + force_magnitude;

hand_forces=hand_forces*load_scaling;
